simulink library "BechamoNasaOpenModels"  (R2024b)
settings: Solver=VariableStepAuto  StartTime=0.0  StopTime=10.0  RelTol=1e-3
values from neighbouring files (symbols this model uses):
  Cl_aileron_wing_1 = Cl_mat.Claileron_wing.axes1.value    [setupMavrik.m]
  Cl_aileron_wing_2 = Cl_mat.Claileron_wing.axes2.value    [setupMavrik.m]
  Cl_aileron_wing_3 = Cl_mat.Claileron_wing.axes3.value    [setupMavrik.m]
  Cl_aileron_wing_val = Cl_mat.Claileron_wing.value    [setupMavrik.m]
  Cl_elevator_tail_1 = Cl_mat.Clelevator_tail.axes1.value    [setupMavrik.m]
  Cl_elevator_tail_2 = Cl_mat.Clelevator_tail.axes2.value    [setupMavrik.m]
  Cl_elevator_tail_3 = Cl_mat.Clelevator_tail.axes3.value    [setupMavrik.m]
  Cl_elevator_tail_val = Cl_mat.Clelevator_tail.value    [setupMavrik.m]
  Cl_flap_wing_1 = Cl_mat.Clflap_wing.axes1.value    [setupMavrik.m]
  Cl_flap_wing_2 = Cl_mat.Clflap_wing.axes2.value    [setupMavrik.m]
  Cl_flap_wing_3 = Cl_mat.Clflap_wing.axes3.value    [setupMavrik.m]
  Cl_flap_wing_val = Cl_mat.Clflap_wing.value    [setupMavrik.m]
  Cl_hover_fuse_1 = Cl_mat.Clhover_fuse.axes1.value    [setupMavrik.m]
  Cl_hover_fuse_2 = Cl_mat.Clhover_fuse.axes2.value    [setupMavrik.m]
  Cl_hover_fuse_3 = Cl_mat.Clhover_fuse.axes3.value    [setupMavrik.m]
  Cl_hover_fuse_val = Cl_mat.Clhover_fuse.value    [setupMavrik.m]
  Cl_rudder_tail_1 = Cl_mat.Clrudder_tail.axes1.value    [setupMavrik.m]
  Cl_rudder_tail_2 = Cl_mat.Clrudder_tail.axes2.value    [setupMavrik.m]
  Cl_rudder_tail_3 = Cl_mat.Clrudder_tail.axes3.value    [setupMavrik.m]
  Cl_rudder_tail_val = Cl_mat.Clrudder_tail.value    [setupMavrik.m]
  Cl_tail_1 = Cl_mat.Cltail.axes1.value    [setupMavrik.m]
  Cl_tail_2 = Cl_mat.Cltail.axes2.value    [setupMavrik.m]
  Cl_tail_3 = Cl_mat.Cltail.axes3.value    [setupMavrik.m]
  Cl_tail_damp_p_1 = Cl_mat.Cltail_damp_p.axes1.value    [setupMavrik.m]
  Cl_tail_damp_p_2 = Cl_mat.Cltail_damp_p.axes2.value    [setupMavrik.m]
  Cl_tail_damp_p_3 = Cl_mat.Cltail_damp_p.axes3.value    [setupMavrik.m]
  Cl_tail_damp_p_val = Cl_mat.Cltail_damp_p.value    [setupMavrik.m]
  Cl_tail_damp_q_1 = Cl_mat.Cltail_damp_q.axes1.value    [setupMavrik.m]
  Cl_tail_damp_q_2 = Cl_mat.Cltail_damp_q.axes2.value    [setupMavrik.m]
  Cl_tail_damp_q_3 = Cl_mat.Cltail_damp_q.axes3.value    [setupMavrik.m]
  Cl_tail_damp_q_val = Cl_mat.Cltail_damp_q.value    [setupMavrik.m]
  Cl_tail_damp_r_1 = Cl_mat.Cltail_damp_r.axes1.value    [setupMavrik.m]
  Cl_tail_damp_r_2 = Cl_mat.Cltail_damp_r.axes2.value    [setupMavrik.m]
  Cl_tail_damp_r_3 = Cl_mat.Cltail_damp_r.axes3.value    [setupMavrik.m]
  Cl_tail_damp_r_val = Cl_mat.Cltail_damp_r.value    [setupMavrik.m]
  Cl_tail_val = Cl_mat.Cltail.value    [setupMavrik.m]
  Cl_wing_1 = Cl_mat.Clwing.axes1.value    [setupMavrik.m]
  Cl_wing_2 = Cl_mat.Clwing.axes2.value    [setupMavrik.m]
  Cl_wing_3 = Cl_mat.Clwing.axes3.value    [setupMavrik.m]
  Cl_wing_damp_p_1 = Cl_mat.Clwing_damp_p.axes1.value    [setupMavrik.m]
  Cl_wing_damp_p_2 = Cl_mat.Clwing_damp_p.axes2.value    [setupMavrik.m]
  Cl_wing_damp_p_3 = Cl_mat.Clwing_damp_p.axes3.value    [setupMavrik.m]
  Cl_wing_damp_p_val = Cl_mat.Clwing_damp_p.value    [setupMavrik.m]
  Cl_wing_damp_q_1 = Cl_mat.Clwing_damp_q.axes1.value    [setupMavrik.m]
  Cl_wing_damp_q_2 = Cl_mat.Clwing_damp_q.axes2.value    [setupMavrik.m]
  Cl_wing_damp_q_3 = Cl_mat.Clwing_damp_q.axes3.value    [setupMavrik.m]
  Cl_wing_damp_q_val = Cl_mat.Clwing_damp_q.value    [setupMavrik.m]
  Cl_wing_damp_r_1 = Cl_mat.Clwing_damp_r.axes1.value    [setupMavrik.m]
  Cl_wing_damp_r_2 = Cl_mat.Clwing_damp_r.axes2.value    [setupMavrik.m]
  Cl_wing_damp_r_3 = Cl_mat.Clwing_damp_r.axes3.value    [setupMavrik.m]
  Cl_wing_damp_r_val = Cl_mat.Clwing_damp_r.value    [setupMavrik.m]
  Cl_wing_val = Cl_mat.Clwing.value    [setupMavrik.m]
  Cm_aileron_wing_1 = Cm_mat.Cmaileron_wing.axes1.value    [setupMavrik.m]
  Cm_aileron_wing_2 = Cm_mat.Cmaileron_wing.axes2.value    [setupMavrik.m]
  Cm_aileron_wing_3 = Cm_mat.Cmaileron_wing.axes3.value    [setupMavrik.m]
  Cm_aileron_wing_val = Cm_mat.Cmaileron_wing.value    [setupMavrik.m]
  Cm_elevator_tail_1 = Cm_mat.Cmelevator_tail.axes1.value    [setupMavrik.m]
  Cm_elevator_tail_2 = Cm_mat.Cmelevator_tail.axes2.value    [setupMavrik.m]
  Cm_elevator_tail_3 = Cm_mat.Cmelevator_tail.axes3.value    [setupMavrik.m]
  Cm_elevator_tail_val = Cm_mat.Cmelevator_tail.value    [setupMavrik.m]
  Cm_flap_wing_1 = Cm_mat.Cmflap_wing.axes1.value    [setupMavrik.m]
  Cm_flap_wing_2 = Cm_mat.Cmflap_wing.axes2.value    [setupMavrik.m]
  Cm_flap_wing_3 = Cm_mat.Cmflap_wing.axes3.value    [setupMavrik.m]
  Cm_flap_wing_val = Cm_mat.Cmflap_wing.value    [setupMavrik.m]
  Cm_hover_fuse_1 = Cm_mat.Cmhover_fuse.axes1.value    [setupMavrik.m]
  Cm_hover_fuse_2 = Cm_mat.Cmhover_fuse.axes2.value    [setupMavrik.m]
  Cm_hover_fuse_3 = Cm_mat.Cmhover_fuse.axes3.value    [setupMavrik.m]
  Cm_hover_fuse_val = Cm_mat.Cmhover_fuse.value    [setupMavrik.m]
  Cm_rudder_tail_1 = Cm_mat.Cmrudder_tail.axes1.value    [setupMavrik.m]
  Cm_rudder_tail_2 = Cm_mat.Cmrudder_tail.axes2.value    [setupMavrik.m]
  Cm_rudder_tail_3 = Cm_mat.Cmrudder_tail.axes3.value    [setupMavrik.m]
  Cm_rudder_tail_val = Cm_mat.Cmrudder_tail.value    [setupMavrik.m]
  Cm_tail_1 = Cm_mat.Cmtail.axes1.value    [setupMavrik.m]
  Cm_tail_2 = Cm_mat.Cmtail.axes2.value    [setupMavrik.m]
  Cm_tail_3 = Cm_mat.Cmtail.axes3.value    [setupMavrik.m]
  Cm_tail_damp_p_1 = Cm_mat.Cmtail_damp_p.axes1.value    [setupMavrik.m]
  Cm_tail_damp_p_2 = Cm_mat.Cmtail_damp_p.axes2.value    [setupMavrik.m]
  Cm_tail_damp_p_3 = Cm_mat.Cmtail_damp_p.axes3.value    [setupMavrik.m]
  Cm_tail_damp_p_val = Cm_mat.Cmtail_damp_p.value    [setupMavrik.m]
  Cm_tail_damp_q_1 = Cm_mat.Cmtail_damp_q.axes1.value    [setupMavrik.m]
  Cm_tail_damp_q_2 = Cm_mat.Cmtail_damp_q.axes2.value    [setupMavrik.m]
  Cm_tail_damp_q_3 = Cm_mat.Cmtail_damp_q.axes3.value    [setupMavrik.m]
  Cm_tail_damp_q_val = Cm_mat.Cmtail_damp_q.value    [setupMavrik.m]
  Cm_tail_damp_r_1 = Cm_mat.Cmtail_damp_r.axes1.value    [setupMavrik.m]
  Cm_tail_damp_r_2 = Cm_mat.Cmtail_damp_r.axes2.value    [setupMavrik.m]
  Cm_tail_damp_r_3 = Cm_mat.Cmtail_damp_r.axes3.value    [setupMavrik.m]
  Cm_tail_damp_r_val = Cm_mat.Cmtail_damp_r.value    [setupMavrik.m]
  Cm_tail_val = Cm_mat.Cmtail.value    [setupMavrik.m]
  Cm_wing_1 = Cm_mat.Cmwing.axes1.value    [setupMavrik.m]
  Cm_wing_2 = Cm_mat.Cmwing.axes2.value    [setupMavrik.m]
  Cm_wing_3 = Cm_mat.Cmwing.axes3.value    [setupMavrik.m]
  Cm_wing_damp_p_1 = Cm_mat.Cmwing_damp_p.axes1.value    [setupMavrik.m]
  Cm_wing_damp_p_2 = Cm_mat.Cmwing_damp_p.axes2.value    [setupMavrik.m]
  Cm_wing_damp_p_3 = Cm_mat.Cmwing_damp_p.axes3.value    [setupMavrik.m]
  Cm_wing_damp_p_val = Cm_mat.Cmwing_damp_p.value    [setupMavrik.m]
  Cm_wing_damp_q_1 = Cm_mat.Cmwing_damp_q.axes1.value    [setupMavrik.m]
  Cm_wing_damp_q_2 = Cm_mat.Cmwing_damp_q.axes2.value    [setupMavrik.m]
  Cm_wing_damp_q_3 = Cm_mat.Cmwing_damp_q.axes3.value    [setupMavrik.m]
  Cm_wing_damp_q_val = Cm_mat.Cmwing_damp_q.value    [setupMavrik.m]
  Cm_wing_damp_r_1 = Cm_mat.Cmwing_damp_r.axes1.value    [setupMavrik.m]
  Cm_wing_damp_r_2 = Cm_mat.Cmwing_damp_r.axes2.value    [setupMavrik.m]
  Cm_wing_damp_r_3 = Cm_mat.Cmwing_damp_r.axes3.value    [setupMavrik.m]
  Cm_wing_damp_r_val = Cm_mat.Cmwing_damp_r.value    [setupMavrik.m]
  Cm_wing_val = Cm_mat.Cmwing.value    [setupMavrik.m]
  Cn_aileron_wing_1 = Cn_mat.Cnaileron_wing.axes1.value    [setupMavrik.m]
  Cn_aileron_wing_2 = Cn_mat.Cnaileron_wing.axes2.value    [setupMavrik.m]
  Cn_aileron_wing_3 = Cn_mat.Cnaileron_wing.axes3.value    [setupMavrik.m]
  Cn_aileron_wing_val = Cn_mat.Cnaileron_wing.value    [setupMavrik.m]
  Cn_elevator_tail_1 = Cn_mat.Cnelevator_tail.axes1.value    [setupMavrik.m]
  Cn_elevator_tail_2 = Cn_mat.Cnelevator_tail.axes2.value    [setupMavrik.m]
  Cn_elevator_tail_3 = Cn_mat.Cnelevator_tail.axes3.value    [setupMavrik.m]
  Cn_elevator_tail_val = Cn_mat.Cnelevator_tail.value    [setupMavrik.m]
  Cn_flap_wing_1 = Cn_mat.Cnflap_wing.axes1.value    [setupMavrik.m]
  Cn_flap_wing_2 = Cn_mat.Cnflap_wing.axes2.value    [setupMavrik.m]
  Cn_flap_wing_3 = Cn_mat.Cnflap_wing.axes3.value    [setupMavrik.m]
  Cn_flap_wing_val = Cn_mat.Cnflap_wing.value    [setupMavrik.m]
  Cn_hover_fuse_1 = Cn_mat.Cnhover_fuse.axes1.value    [setupMavrik.m]
  Cn_hover_fuse_2 = Cn_mat.Cnhover_fuse.axes2.value    [setupMavrik.m]
  Cn_hover_fuse_3 = Cn_mat.Cnhover_fuse.axes3.value    [setupMavrik.m]
  Cn_hover_fuse_val = Cn_mat.Cnhover_fuse.value    [setupMavrik.m]
  ... (+319 more)
libraries: matrix_library x15, sharedtransform x2, $bdroot x1, shared6dof x1
(part 4 of 19)

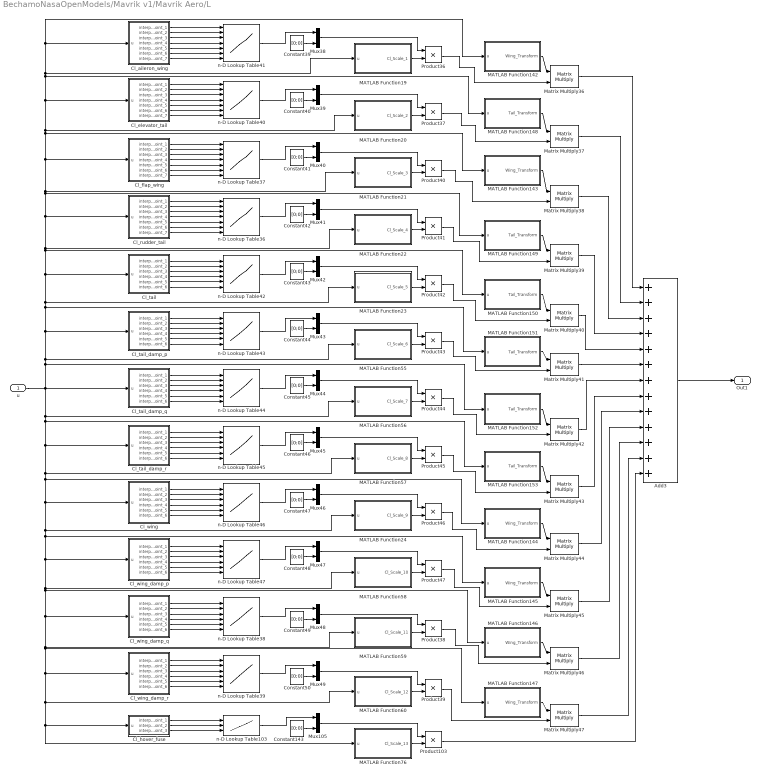
== system BechamoNasaOpenModels/Mavrik v1/Mavrik Aero/L ==
  u : Inport
  Add3 : Sum  Inputs=+++++++++++++
  Cl_aileron_wing : MATLAB Function  TreatAsAtomicUnit=on
  Cl_elevator_tail : MATLAB Function  TreatAsAtomicUnit=on
  Cl_flap_wing : MATLAB Function  TreatAsAtomicUnit=on
  Cl_hover_fuse : MATLAB Function  TreatAsAtomicUnit=on
  Cl_rudder_tail : MATLAB Function  TreatAsAtomicUnit=on
  Cl_tail : MATLAB Function  TreatAsAtomicUnit=on
  Cl_tail_damp_p : MATLAB Function  TreatAsAtomicUnit=on
  Cl_tail_damp_q : MATLAB Function  TreatAsAtomicUnit=on
  Cl_tail_damp_r : MATLAB Function  TreatAsAtomicUnit=on
  Cl_wing : MATLAB Function  TreatAsAtomicUnit=on
  Cl_wing_damp_p : MATLAB Function  TreatAsAtomicUnit=on
  Cl_wing_damp_q : MATLAB Function  TreatAsAtomicUnit=on
  Cl_wing_damp_r : MATLAB Function  TreatAsAtomicUnit=on
  Constant{39..50,143} (13 alike) : Constant  Value=[0;0]
  MATLAB Function142 : MATLAB Function  TreatAsAtomicUnit=on
  MATLAB Function143 : MATLAB Function  TreatAsAtomicUnit=on
  MATLAB Function144 : MATLAB Function  TreatAsAtomicUnit=on
  MATLAB Function145 : MATLAB Function  TreatAsAtomicUnit=on
  MATLAB Function146 : MATLAB Function  TreatAsAtomicUnit=on
  MATLAB Function147 : MATLAB Function  TreatAsAtomicUnit=on
  MATLAB Function148 : MATLAB Function  TreatAsAtomicUnit=on
  MATLAB Function149 : MATLAB Function  TreatAsAtomicUnit=on
  MATLAB Function150 : MATLAB Function  TreatAsAtomicUnit=on
  MATLAB Function151 : MATLAB Function  TreatAsAtomicUnit=on
  MATLAB Function152 : MATLAB Function  TreatAsAtomicUnit=on
  MATLAB Function153 : MATLAB Function  TreatAsAtomicUnit=on
  MATLAB Function19 : MATLAB Function  TreatAsAtomicUnit=on
  MATLAB Function20 : MATLAB Function  TreatAsAtomicUnit=on
  MATLAB Function21 : MATLAB Function  TreatAsAtomicUnit=on
  MATLAB Function22 : MATLAB Function  TreatAsAtomicUnit=on
  MATLAB Function23 : MATLAB Function  TreatAsAtomicUnit=on
  MATLAB Function24 : MATLAB Function  TreatAsAtomicUnit=on
  MATLAB Function55 : MATLAB Function  TreatAsAtomicUnit=on
  MATLAB Function56 : MATLAB Function  TreatAsAtomicUnit=on
  MATLAB Function57 : MATLAB Function  TreatAsAtomicUnit=on
  MATLAB Function58 : MATLAB Function  TreatAsAtomicUnit=on
  MATLAB Function59 : MATLAB Function  TreatAsAtomicUnit=on
  MATLAB Function60 : MATLAB Function  TreatAsAtomicUnit=on
  MATLAB Function76 : MATLAB Function  TreatAsAtomicUnit=on
  Matrix Multiply{36..47} (12 alike) : Product  Multiplication=Matrix(*)
  Mux{38..49,105} (13 alike) : Mux  Inputs=2
  Product{36..47,103} (13 alike) : Product
  n-D Lookup Table103 : Lookup_n-D  NumberOfTableDimensions=3  BreakpointsForDimension1=Cl_hover_fuse_1  BreakpointsForDimension2=Cl_hover_fuse_2  BreakpointsForDimension3=Cl_hover_fuse_3  BreakpointsForDimension4=CX_wing_damp_r_4  BreakpointsForDimension5=CX_wing_damp_r_5  BreakpointsForDimension6=CX_wing_damp_r_6  BreakpointsForDimension7=CX_flap_wing_7  Table=Cl_hover_fuse_val  InternalRulePriority=Speed  OutDataTypeStr=Inherit: Inherit via back propagation  RndMeth=Simplest
      settings: InputPortMap=u0,u1,u2
  n-D Lookup Table36 : Lookup_n-D  NumberOfTableDimensions=7  BreakpointsForDimension1=Cl_rudder_tail_1  BreakpointsForDimension2=Cl_rudder_tail_2  BreakpointsForDimension3=Cl_rudder_tail_3  BreakpointsForDimension4=Cl_rudder_tail_4  BreakpointsForDimension5=Cl_rudder_tail_5  BreakpointsForDimension6=Cl_rudder_tail_6  BreakpointsForDimension7=Cl_rudder_tail_7  Table=Cl_rudder_tail_val  InternalRulePriority=Speed  OutDataTypeStr=Inherit: Inherit via back propagation  RndMeth=Simplest
      settings: InputPortMap=u0,u1,u2,u3,u4,u5,u6
  n-D Lookup Table37 : Lookup_n-D  NumberOfTableDimensions=7  BreakpointsForDimension1=Cl_flap_wing_1  BreakpointsForDimension2=Cl_flap_wing_2  BreakpointsForDimension3=Cl_flap_wing_3  BreakpointsForDimension4=Cl_flap_wing_4  BreakpointsForDimension5=Cl_flap_wing_5  BreakpointsForDimension6=Cl_flap_wing_6  BreakpointsForDimension7=Cl_flap_wing_7  Table=Cl_flap_wing_val  InternalRulePriority=Speed  OutDataTypeStr=Inherit: Inherit via back propagation  RndMeth=Simplest
      settings: InputPortMap=u0,u1,u2,u3,u4,u5,u6
  n-D Lookup Table38 : Lookup_n-D  NumberOfTableDimensions=6  BreakpointsForDimension1=Cl_wing_damp_q_1  BreakpointsForDimension2=Cl_wing_damp_q_2  BreakpointsForDimension3=Cl_wing_damp_q_3  BreakpointsForDimension4=Cl_wing_damp_q_4  BreakpointsForDimension5=Cl_wing_damp_q_5  BreakpointsForDimension6=Cl_wing_damp_q_6  BreakpointsForDimension7=CX_flap_wing_7  Table=Cl_wing_damp_q_val  InternalRulePriority=Speed  OutDataTypeStr=Inherit: Inherit via back propagation  RndMeth=Simplest
      settings: InputPortMap=u0,u1,u2,u3,u4,u5
  n-D Lookup Table39 : Lookup_n-D  NumberOfTableDimensions=6  BreakpointsForDimension1=Cl_wing_damp_r_1  BreakpointsForDimension2=Cl_wing_damp_r_2  BreakpointsForDimension3=Cl_wing_damp_r_3  BreakpointsForDimension4=Cl_wing_damp_r_4  BreakpointsForDimension5=Cl_wing_damp_r_5  BreakpointsForDimension6=Cl_wing_damp_r_6  BreakpointsForDimension7=CX_flap_wing_7  Table=Cl_wing_damp_r_val  InternalRulePriority=Speed  OutDataTypeStr=Inherit: Inherit via back propagation  RndMeth=Simplest
      settings: InputPortMap=u0,u1,u2,u3,u4,u5
  n-D Lookup Table40 : Lookup_n-D  NumberOfTableDimensions=7  BreakpointsForDimension1=Cl_elevator_tail_1  BreakpointsForDimension2=Cl_elevator_tail_2  BreakpointsForDimension3=Cl_elevator_tail_3  BreakpointsForDimension4=Cl_elevator_tail_4  BreakpointsForDimension5=Cl_elevator_tail_5  BreakpointsForDimension6=Cl_elevator_tail_6  BreakpointsForDimension7=Cl_elevator_tail_7  Table=Cl_elevator_tail_val  InternalRulePriority=Speed  OutDataTypeStr=Inherit: Inherit via back propagation  RndMeth=Simplest
      settings: InputPortMap=u0,u1,u2,u3,u4,u5,u6
  n-D Lookup Table41 : Lookup_n-D  NumberOfTableDimensions=7  BreakpointsForDimension1=Cl_aileron_wing_1  BreakpointsForDimension2=Cl_aileron_wing_2  BreakpointsForDimension3=Cl_aileron_wing_3  BreakpointsForDimension4=Cl_aileron_wing_4  BreakpointsForDimension5=Cl_aileron_wing_5  BreakpointsForDimension6=Cl_aileron_wing_6  BreakpointsForDimension7=Cl_aileron_wing_7  Table=Cl_aileron_wing_val  InternalRulePriority=Speed  OutDataTypeStr=Inherit: Inherit via back propagation  RndMeth=Simplest
      settings: InputPortMap=u0,u1,u2,u3,u4,u5,u6
  n-D Lookup Table42 : Lookup_n-D  NumberOfTableDimensions=6  BreakpointsForDimension1=Cl_tail_1  BreakpointsForDimension2=Cl_tail_2  BreakpointsForDimension3=Cl_tail_3  BreakpointsForDimension4=Cl_tail_4  BreakpointsForDimension5=Cl_tail_5  BreakpointsForDimension6=Cl_tail_6  BreakpointsForDimension7=CX_tail_7  Table=Cl_tail_val  InternalRulePriority=Speed  OutDataTypeStr=Inherit: Inherit via back propagation  RndMeth=Simplest
      settings: InputPortMap=u0,u1,u2,u3,u4,u5
  n-D Lookup Table43 : Lookup_n-D  NumberOfTableDimensions=6  BreakpointsForDimension1=Cl_tail_damp_p_1  BreakpointsForDimension2=Cl_tail_damp_p_2  BreakpointsForDimension3=Cl_tail_damp_p_3  BreakpointsForDimension4=Cl_tail_damp_p_4  BreakpointsForDimension5=Cl_tail_damp_p_5  BreakpointsForDimension6=Cl_tail_damp_p_6  BreakpointsForDimension7=CX_tail_7  Table=Cl_tail_damp_p_val  InternalRulePriority=Speed  OutDataTypeStr=Inherit: Inherit via back propagation  RndMeth=Simplest
      settings: InputPortMap=u0,u1,u2,u3,u4,u5
  n-D Lookup Table44 : Lookup_n-D  NumberOfTableDimensions=6  BreakpointsForDimension1=Cl_tail_damp_q_1  BreakpointsForDimension2=Cl_tail_damp_q_2  BreakpointsForDimension3=Cl_tail_damp_q_3  BreakpointsForDimension4=Cl_tail_damp_q_4  BreakpointsForDimension5=Cl_tail_damp_q_5  BreakpointsForDimension6=Cl_tail_damp_q_6  BreakpointsForDimension7=CX_tail_7  Table=Cl_tail_damp_q_val  InternalRulePriority=Speed  OutDataTypeStr=Inherit: Inherit via back propagation  RndMeth=Simplest
      settings: InputPortMap=u0,u1,u2,u3,u4,u5
  n-D Lookup Table45 : Lookup_n-D  NumberOfTableDimensions=6  BreakpointsForDimension1=Cl_tail_damp_r_1  BreakpointsForDimension2=Cl_tail_damp_r_2  BreakpointsForDimension3=Cl_tail_damp_r_3  BreakpointsForDimension4=Cl_tail_damp_r_4  BreakpointsForDimension5=Cl_tail_damp_r_5  BreakpointsForDimension6=Cl_tail_damp_r_6  BreakpointsForDimension7=CX_tail_7  Table=Cl_tail_damp_r_val  InternalRulePriority=Speed  OutDataTypeStr=Inherit: Inherit via back propagation  RndMeth=Simplest
      settings: InputPortMap=u0,u1,u2,u3,u4,u5
  n-D Lookup Table46 : Lookup_n-D  NumberOfTableDimensions=6  BreakpointsForDimension1=Cl_wing_1  BreakpointsForDimension2=Cl_wing_2  BreakpointsForDimension3=Cl_wing_3  BreakpointsForDimension4=Cl_wing_4  BreakpointsForDimension5=Cl_wing_5  BreakpointsForDimension6=Cl_wing_6  BreakpointsForDimension7=CX_flap_wing_7  Table=Cl_wing_val  InternalRulePriority=Speed  OutDataTypeStr=Inherit: Inherit via back propagation  RndMeth=Simplest
      settings: InputPortMap=u0,u1,u2,u3,u4,u5
  n-D Lookup Table47 : Lookup_n-D  NumberOfTableDimensions=6  BreakpointsForDimension1=Cl_wing_damp_p_1  BreakpointsForDimension2=Cl_wing_damp_p_2  BreakpointsForDimension3=Cl_wing_damp_p_3  BreakpointsForDimension4=Cl_wing_damp_p_4  BreakpointsForDimension5=Cl_wing_damp_p_5  BreakpointsForDimension6=Cl_wing_damp_p_6  BreakpointsForDimension7=CX_flap_wing_7  Table=Cl_wing_damp_p_val  InternalRulePriority=Speed  OutDataTypeStr=Inherit: Inherit via back propagation  RndMeth=Simplest
      settings: InputPortMap=u0,u1,u2,u3,u4,u5
  Out1 : Outport
  wires:
  Cl_hover_fuse/3(interp_point_3) -> n-D Lookup Table103/3
  Cl_wing_damp_q/1(interp_point_1) -> n-D Lookup Table38/1
  Add3/1 -> Out1/1
  Cl_wing/3(interp_point_3) -> n-D Lookup Table46/3
  MATLAB Function57/1(Cl_Scale_8) -> Product45/2
  Cl_tail_damp_q/3(interp_point_3) -> n-D Lookup Table44/3
  Matrix Multiply46/1 -> Add3/11
  Cl_elevator_tail/5(interp_point_5) -> n-D Lookup Table40/5
  MATLAB Function153/1(Tail_Transform) -> Matrix Multiply43/1
  Matrix Multiply40/1 -> Add3/5
  Cl_rudder_tail/4(interp_point_4) -> n-D Lookup Table36/4
  Cl_tail_damp_r/1(interp_point_1) -> n-D Lookup Table45/1
  Matrix Multiply38/1 -> Add3/3
  Matrix Multiply37/1 -> Add3/2
  Cl_tail_damp_p/5(interp_point_5) -> n-D Lookup Table43/5
  Mux48/1 -> Product38/1
  Cl_wing_damp_p/6(interp_point_6) -> n-D Lookup Table47/6
  Cl_wing_damp_q/4(interp_point_4) -> n-D Lookup Table38/4
  MATLAB Function21/1(Cl_Scale_3) -> Product40/2
  Cl_wing_damp_p/5(interp_point_5) -> n-D Lookup Table47/5
  Mux44/1 -> Product44/1
  Matrix Multiply36/1 -> Add3/1
  Cl_rudder_tail/5(interp_point_5) -> n-D Lookup Table36/5
  Product44/1 -> Matrix Multiply42/2
  Mux41/1 -> Product41/1
  Cl_elevator_tail/4(interp_point_4) -> n-D Lookup Table40/4
  Cl_rudder_tail/2(interp_point_2) -> n-D Lookup Table36/2
  Cl_wing_damp_p/3(interp_point_3) -> n-D Lookup Table47/3
  Cl_elevator_tail/2(interp_point_2) -> n-D Lookup Table40/2
  Mux42/1 -> Product42/1
  Cl_tail/3(interp_point_3) -> n-D Lookup Table42/3
  Cl_wing/5(interp_point_5) -> n-D Lookup Table46/5
  Cl_tail_damp_r/5(interp_point_5) -> n-D Lookup Table45/5
  Cl_wing/2(interp_point_2) -> n-D Lookup Table46/2
  Cl_tail_damp_q/4(interp_point_4) -> n-D Lookup Table44/4
  Cl_flap_wing/3(interp_point_3) -> n-D Lookup Table37/3
  Mux47/1 -> Product47/1
  Cl_tail/5(interp_point_5) -> n-D Lookup Table42/5
  Product103/1 -> Add3/13
  Cl_elevator_tail/1(interp_point_1) -> n-D Lookup Table40/1
  Cl_tail_damp_q/1(interp_point_1) -> n-D Lookup Table44/1
  Constant47/1 -> Mux46/2
  Cl_wing_damp_r/3(interp_point_3) -> n-D Lookup Table39/3
  Cl_wing_damp_r/4(interp_point_4) -> n-D Lookup Table39/4
  Cl_tail_damp_q/2(interp_point_2) -> n-D Lookup Table44/2
  MATLAB Function24/1(Cl_Scale_9) -> Product46/2
  Cl_tail/6(interp_point_6) -> n-D Lookup Table42/6
  Cl_rudder_tail/3(interp_point_3) -> n-D Lookup Table36/3
  MATLAB Function142/1(Wing_Transform) -> Matrix Multiply36/1
  Cl_hover_fuse/1(interp_point_1) -> n-D Lookup Table103/1
  Cl_wing/1(interp_point_1) -> n-D Lookup Table46/1
  Cl_wing_damp_q/6(interp_point_6) -> n-D Lookup Table38/6
  Cl_rudder_tail/7(interp_point_7) -> n-D Lookup Table36/7
  Cl_aileron_wing/1(interp_point_1) -> n-D Lookup Table41/1
  Cl_wing/6(interp_point_6) -> n-D Lookup Table46/6
  n-D Lookup Table44/1 -> Mux44/1
  Cl_elevator_tail/7(interp_point_7) -> n-D Lookup Table40/7
  Cl_tail_damp_p/6(interp_point_6) -> n-D Lookup Table43/6
  Constant42/1 -> Mux41/2
  u/1 -> MATLAB Function56/1(u), MATLAB Function153/1(u), Cl_tail_damp_r/1(u), MATLAB Function57/1(u), MATLAB Function144/1(u), Cl_wing/1(u), MATLAB Function24/1(u), MATLAB Function145/1(u), Cl_wing_damp_p/1(u), MATLAB Function58/1(u), MATLAB Function146/1(u), Cl_wing_damp_q/1(u), MATLAB Function59/1(u), Cl_wing_damp_r/1(u), MATLAB Function60/1(u), Cl_hover_fuse/1(u), MATLAB Function76/1(u), MATLAB Function147/1(u), MATLAB Function152/1(u), MATLAB Function55/1(u), Cl_tail_damp_p/1(u), MATLAB Function151/1(u), MATLAB Function23/1(u), Cl_tail/1(u), MATLAB Function150/1(u), MATLAB Function22/1(u), Cl_rudder_tail/1(u), MATLAB Function149/1(u), MATLAB Function21/1(u), Cl_flap_wing/1(u), MATLAB Function143/1(u), MATLAB Function20/1(u), Cl_elevator_tail/1(u), MATLAB Function148/1(u), Cl_aileron_wing/1(u), MATLAB Function142/1(u), MATLAB Function19/1(u), Cl_tail_damp_q/1(u)
  Cl_wing_damp_r/5(interp_point_5) -> n-D Lookup Table39/5
  Cl_hover_fuse/2(interp_point_2) -> n-D Lookup Table103/2
  Cl_aileron_wing/3(interp_point_3) -> n-D Lookup Table41/3
  MATLAB Function147/1(Wing_Transform) -> Matrix Multiply47/1
  Cl_flap_wing/1(interp_point_1) -> n-D Lookup Table37/1
  Constant41/1 -> Mux40/2
  Cl_tail_damp_p/3(interp_point_3) -> n-D Lookup Table43/3
  Cl_tail_damp_p/4(interp_point_4) -> n-D Lookup Table43/4
  n-D Lookup Table103/1 -> Mux105/1
  Cl_tail_damp_r/4(interp_point_4) -> n-D Lookup Table45/4
  n-D Lookup Table46/1 -> Mux46/1
  Cl_tail_damp_q/5(interp_point_5) -> n-D Lookup Table44/5
  Cl_tail_damp_r/6(interp_point_6) -> n-D Lookup Table45/6
  Cl_flap_wing/5(interp_point_5) -> n-D Lookup Table37/5
  Cl_tail_damp_r/2(interp_point_2) -> n-D Lookup Table45/2
  Cl_wing/4(interp_point_4) -> n-D Lookup Table46/4
  Constant50/1 -> Mux49/2
  MATLAB Function60/1(Cl_Scale_12) -> Product39/2
  MATLAB Function76/1(Cl_Scale_13) -> Product103/2
  Cl_wing_damp_p/2(interp_point_2) -> n-D Lookup Table47/2
  Cl_wing_damp_p/1(interp_point_1) -> n-D Lookup Table47/1
  Matrix Multiply39/1 -> Add3/4
  MATLAB Function59/1(Cl_Scale_11) -> Product38/2
  Cl_aileron_wing/4(interp_point_4) -> n-D Lookup Table41/4
  Cl_wing_damp_r/1(interp_point_1) -> n-D Lookup Table39/1
  Cl_wing_damp_r/6(interp_point_6) -> n-D Lookup Table39/6
  Cl_tail/4(interp_point_4) -> n-D Lookup Table42/4
  MATLAB Function145/1(Wing_Transform) -> Matrix Multiply45/1
  MATLAB Function144/1(Wing_Transform) -> Matrix Multiply44/1
  Cl_flap_wing/6(interp_point_6) -> n-D Lookup Table37/6
  Cl_flap_wing/4(interp_point_4) -> n-D Lookup Table37/4
  Mux45/1 -> Product45/1
  Cl_tail_damp_q/6(interp_point_6) -> n-D Lookup Table44/6
  n-D Lookup Table42/1 -> Mux42/1
  MATLAB Function151/1(Tail_Transform) -> Matrix Multiply41/1
  Matrix Multiply45/1 -> Add3/10
  Cl_tail/2(interp_point_2) -> n-D Lookup Table42/2
  Constant143/1 -> Mux105/2
  Mux39/1 -> Product37/1
  Product42/1 -> Matrix Multiply40/2
  Cl_flap_wing/2(interp_point_2) -> n-D Lookup Table37/2
  Cl_tail/1(interp_point_1) -> n-D Lookup Table42/1
  Product38/1 -> Matrix Multiply46/2
  Cl_aileron_wing/7(interp_point_7) -> n-D Lookup Table41/7
  MATLAB Function20/1(Cl_Scale_2) -> Product37/2
  Product41/1 -> Matrix Multiply39/2
  MATLAB Function146/1(Wing_Transform) -> Matrix Multiply46/1
  Cl_wing_damp_q/5(interp_point_5) -> n-D Lookup Table38/5
  MATLAB Function23/1(Cl_Scale_5) -> Product42/2
  MATLAB Function148/1(Tail_Transform) -> Matrix Multiply37/1
  n-D Lookup Table39/1 -> Mux49/1
  Product46/1 -> Matrix Multiply44/2
  Matrix Multiply44/1 -> Add3/9
  Matrix Multiply47/1 -> Add3/12
  Matrix Multiply41/1 -> Add3/6
  Matrix Multiply42/1 -> Add3/7
  n-D Lookup Table43/1 -> Mux43/1
  n-D Lookup Table41/1 -> Mux38/1
  Constant44/1 -> Mux43/2
  n-D Lookup Table45/1 -> Mux45/1
  Constant46/1 -> Mux45/2
  Constant49/1 -> Mux48/2
  n-D Lookup Table47/1 -> Mux47/1
  Constant48/1 -> Mux47/2
  n-D Lookup Table38/1 -> Mux48/1
  Cl_wing_damp_q/2(interp_point_2) -> n-D Lookup Table38/2
  Mux38/1 -> Product36/1
  MATLAB Function149/1(Tail_Transform) -> Matrix Multiply39/1
  n-D Lookup Table40/1 -> Mux39/1
  n-D Lookup Table37/1 -> Mux40/1
  Product39/1 -> Matrix Multiply47/2
  Cl_wing_damp_q/3(interp_point_3) -> n-D Lookup Table38/3
  Cl_tail_damp_p/2(interp_point_2) -> n-D Lookup Table43/2
  Constant39/1 -> Mux38/2
  MATLAB Function56/1(Cl_Scale_7) -> Product44/2
  Constant40/1 -> Mux39/2
  MATLAB Function55/1(Cl_Scale_6) -> Product43/2
  MATLAB Function58/1(Cl_Scale_10) -> Product47/2
  Cl_flap_wing/7(interp_point_7) -> n-D Lookup Table37/7
  Cl_aileron_wing/2(interp_point_2) -> n-D Lookup Table41/2
  Cl_tail_damp_p/1(interp_point_1) -> n-D Lookup Table43/1
  Cl_elevator_tail/6(interp_point_6) -> n-D Lookup Table40/6
  Matrix Multiply43/1 -> Add3/8
  Cl_aileron_wing/6(interp_point_6) -> n-D Lookup Table41/6
  Mux49/1 -> Product39/1
  Mux46/1 -> Product46/1
  Cl_wing_damp_r/2(interp_point_2) -> n-D Lookup Table39/2
  Constant45/1 -> Mux44/2
  Mux40/1 -> Product40/1
  Cl_rudder_tail/6(interp_point_6) -> n-D Lookup Table36/6
  Cl_elevator_tail/3(interp_point_3) -> n-D Lookup Table40/3
  MATLAB Function19/1(Cl_Scale_1) -> Product36/2
  MATLAB Function143/1(Wing_Transform) -> Matrix Multiply38/1
  Mux43/1 -> Product43/1
  MATLAB Function152/1(Tail_Transform) -> Matrix Multiply42/1
  MATLAB Function22/1(Cl_Scale_4) -> Product41/2
  n-D Lookup Table36/1 -> Mux41/1
  Cl_wing_damp_p/4(interp_point_4) -> n-D Lookup Table47/4
  Constant43/1 -> Mux42/2
  Cl_tail_damp_r/3(interp_point_3) -> n-D Lookup Table45/3
  Product36/1 -> Matrix Multiply36/2
  Product37/1 -> Matrix Multiply37/2
  Product43/1 -> Matrix Multiply41/2
  Product40/1 -> Matrix Multiply38/2
  Product47/1 -> Matrix Multiply45/2
  Product45/1 -> Matrix Multiply43/2
  Mux105/1 -> Product103/1
  Cl_rudder_tail/1(interp_point_1) -> n-D Lookup Table36/1
  Cl_aileron_wing/5(interp_point_5) -> n-D Lookup Table41/5
  MATLAB Function150/1(Tail_Transform) -> Matrix Multiply40/1

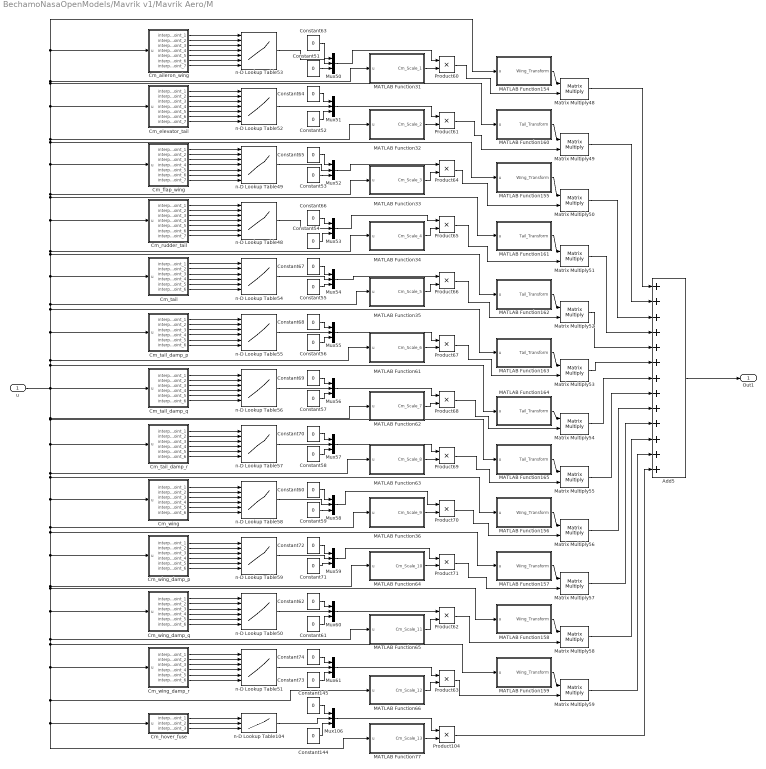
== system BechamoNasaOpenModels/Mavrik v1/Mavrik Aero/M ==
  u : Inport
  Add5 : Sum  Inputs=+++++++++++++
  Cm_aileron_wing : MATLAB Function  TreatAsAtomicUnit=on
  Cm_elevator_tail : MATLAB Function  TreatAsAtomicUnit=on
  Cm_flap_wing : MATLAB Function  TreatAsAtomicUnit=on
  Cm_hover_fuse : MATLAB Function  TreatAsAtomicUnit=on
  Cm_rudder_tail : MATLAB Function  TreatAsAtomicUnit=on
  Cm_tail : MATLAB Function  TreatAsAtomicUnit=on
  Cm_tail_damp_p : MATLAB Function  TreatAsAtomicUnit=on
  Cm_tail_damp_q : MATLAB Function  TreatAsAtomicUnit=on
  Cm_tail_damp_r : MATLAB Function  TreatAsAtomicUnit=on
  Cm_wing : MATLAB Function  TreatAsAtomicUnit=on
  Cm_wing_damp_p : MATLAB Function  TreatAsAtomicUnit=on
  Cm_wing_damp_q : MATLAB Function  TreatAsAtomicUnit=on
  Cm_wing_damp_r : MATLAB Function  TreatAsAtomicUnit=on
  Constant{51..74,144..145} (26 alike) : Constant  Value=0
  MATLAB Function154 : MATLAB Function  TreatAsAtomicUnit=on
  MATLAB Function155 : MATLAB Function  TreatAsAtomicUnit=on
  MATLAB Function156 : MATLAB Function  TreatAsAtomicUnit=on
  MATLAB Function157 : MATLAB Function  TreatAsAtomicUnit=on
  MATLAB Function158 : MATLAB Function  TreatAsAtomicUnit=on
  MATLAB Function159 : MATLAB Function  TreatAsAtomicUnit=on
  MATLAB Function160 : MATLAB Function  TreatAsAtomicUnit=on
  MATLAB Function161 : MATLAB Function  TreatAsAtomicUnit=on
  MATLAB Function162 : MATLAB Function  TreatAsAtomicUnit=on
  MATLAB Function163 : MATLAB Function  TreatAsAtomicUnit=on
  MATLAB Function164 : MATLAB Function  TreatAsAtomicUnit=on
  MATLAB Function165 : MATLAB Function  TreatAsAtomicUnit=on
  MATLAB Function31 : MATLAB Function  TreatAsAtomicUnit=on
  MATLAB Function32 : MATLAB Function  TreatAsAtomicUnit=on
  MATLAB Function33 : MATLAB Function  TreatAsAtomicUnit=on
  MATLAB Function34 : MATLAB Function  TreatAsAtomicUnit=on
  MATLAB Function35 : MATLAB Function  TreatAsAtomicUnit=on
  MATLAB Function36 : MATLAB Function  TreatAsAtomicUnit=on
  MATLAB Function61 : MATLAB Function  TreatAsAtomicUnit=on
  MATLAB Function62 : MATLAB Function  TreatAsAtomicUnit=on
  MATLAB Function63 : MATLAB Function  TreatAsAtomicUnit=on
  MATLAB Function64 : MATLAB Function  TreatAsAtomicUnit=on
  MATLAB Function65 : MATLAB Function  TreatAsAtomicUnit=on
  MATLAB Function66 : MATLAB Function  TreatAsAtomicUnit=on
  MATLAB Function77 : MATLAB Function  TreatAsAtomicUnit=on
  Matrix Multiply{48..59} (12 alike) : Product  Multiplication=Matrix(*)
  Mux{50..61,106} (13 alike) : Mux  Inputs=3
  Product{60..71,104} (13 alike) : Product
  n-D Lookup Table104 : Lookup_n-D  NumberOfTableDimensions=3  BreakpointsForDimension1=Cm_hover_fuse_1  BreakpointsForDimension2=Cm_hover_fuse_2  BreakpointsForDimension3=Cm_hover_fuse_3  BreakpointsForDimension4=CX_wing_damp_r_4  BreakpointsForDimension5=CX_wing_damp_r_5  BreakpointsForDimension6=CX_wing_damp_r_6  BreakpointsForDimension7=CX_flap_wing_7  Table=Cm_hover_fuse_val  InternalRulePriority=Speed  OutDataTypeStr=Inherit: Inherit via back propagation  RndMeth=Simplest
      settings: InputPortMap=u0,u1,u2
  n-D Lookup Table48 : Lookup_n-D  NumberOfTableDimensions=7  BreakpointsForDimension1=Cm_rudder_tail_1  BreakpointsForDimension2=Cm_rudder_tail_2  BreakpointsForDimension3=Cm_rudder_tail_3  BreakpointsForDimension4=Cm_rudder_tail_4  BreakpointsForDimension5=Cm_rudder_tail_5  BreakpointsForDimension6=Cm_rudder_tail_6  BreakpointsForDimension7=Cm_rudder_tail_7  Table=Cm_rudder_tail_val  InternalRulePriority=Speed  OutDataTypeStr=Inherit: Inherit via back propagation  RndMeth=Simplest
      settings: InputPortMap=u0,u1,u2,u3,u4,u5,u6
  n-D Lookup Table49 : Lookup_n-D  NumberOfTableDimensions=7  BreakpointsForDimension1=Cm_flap_wing_1  BreakpointsForDimension2=Cm_flap_wing_2  BreakpointsForDimension3=Cm_flap_wing_3  BreakpointsForDimension4=Cm_flap_wing_4  BreakpointsForDimension5=Cm_flap_wing_5  BreakpointsForDimension6=Cm_flap_wing_6  BreakpointsForDimension7=Cm_flap_wing_7  Table=Cm_flap_wing_val  InternalRulePriority=Speed  OutDataTypeStr=Inherit: Inherit via back propagation  RndMeth=Simplest
      settings: InputPortMap=u0,u1,u2,u3,u4,u5,u6
  n-D Lookup Table50 : Lookup_n-D  NumberOfTableDimensions=6  BreakpointsForDimension1=Cm_wing_damp_q_1  BreakpointsForDimension2=Cm_wing_damp_q_2  BreakpointsForDimension3=Cm_wing_damp_q_3  BreakpointsForDimension4=Cm_wing_damp_q_4  BreakpointsForDimension5=Cm_wing_damp_q_5  BreakpointsForDimension6=Cm_wing_damp_q_6  BreakpointsForDimension7=CX_flap_wing_7  Table=Cm_wing_damp_q_val  InternalRulePriority=Speed  OutDataTypeStr=Inherit: Inherit via back propagation  RndMeth=Simplest
      settings: InputPortMap=u0,u1,u2,u3,u4,u5
  n-D Lookup Table51 : Lookup_n-D  NumberOfTableDimensions=6  BreakpointsForDimension1=Cm_wing_damp_r_1  BreakpointsForDimension2=Cm_wing_damp_r_2  BreakpointsForDimension3=Cm_wing_damp_r_3  BreakpointsForDimension4=Cm_wing_damp_r_4  BreakpointsForDimension5=Cm_wing_damp_r_5  BreakpointsForDimension6=Cm_wing_damp_r_6  BreakpointsForDimension7=CX_flap_wing_7  Table=Cm_wing_damp_r_val  InternalRulePriority=Speed  OutDataTypeStr=Inherit: Inherit via back propagation  RndMeth=Simplest
      settings: InputPortMap=u0,u1,u2,u3,u4,u5
  n-D Lookup Table52 : Lookup_n-D  NumberOfTableDimensions=7  BreakpointsForDimension1=Cm_elevator_tail_1  BreakpointsForDimension2=Cm_elevator_tail_2  BreakpointsForDimension3=Cm_elevator_tail_3  BreakpointsForDimension4=Cm_elevator_tail_4  BreakpointsForDimension5=Cm_elevator_tail_5  BreakpointsForDimension6=Cm_elevator_tail_6  BreakpointsForDimension7=Cm_elevator_tail_7  Table=Cm_elevator_tail_val  InternalRulePriority=Speed  OutDataTypeStr=Inherit: Inherit via back propagation  RndMeth=Simplest
      settings: InputPortMap=u0,u1,u2,u3,u4,u5,u6
  n-D Lookup Table53 : Lookup_n-D  NumberOfTableDimensions=7  BreakpointsForDimension1=Cm_aileron_wing_1  BreakpointsForDimension2=Cm_aileron_wing_2  BreakpointsForDimension3=Cm_aileron_wing_3  BreakpointsForDimension4=Cm_aileron_wing_4  BreakpointsForDimension5=Cm_aileron_wing_5  BreakpointsForDimension6=Cm_aileron_wing_6  BreakpointsForDimension7=Cm_aileron_wing_7  Table=Cm_aileron_wing_val  InternalRulePriority=Speed  OutDataTypeStr=Inherit: Inherit via back propagation  RndMeth=Simplest
      settings: InputPortMap=u0,u1,u2,u3,u4,u5,u6
  n-D Lookup Table54 : Lookup_n-D  NumberOfTableDimensions=6  BreakpointsForDimension1=Cm_tail_1  BreakpointsForDimension2=Cm_tail_2  BreakpointsForDimension3=Cm_tail_3  BreakpointsForDimension4=Cm_tail_4  BreakpointsForDimension5=Cm_tail_5  BreakpointsForDimension6=Cm_tail_6  BreakpointsForDimension7=CX_tail_7  Table=Cm_tail_val  InternalRulePriority=Speed  OutDataTypeStr=Inherit: Inherit via back propagation  RndMeth=Simplest
      settings: InputPortMap=u0,u1,u2,u3,u4,u5
  n-D Lookup Table55 : Lookup_n-D  NumberOfTableDimensions=6  BreakpointsForDimension1=Cm_tail_damp_p_1  BreakpointsForDimension2=Cm_tail_damp_p_2  BreakpointsForDimension3=Cm_tail_damp_p_3  BreakpointsForDimension4=Cm_tail_damp_p_4  BreakpointsForDimension5=Cm_tail_damp_p_5  BreakpointsForDimension6=Cm_tail_damp_p_6  BreakpointsForDimension7=CX_tail_7  Table=Cm_tail_damp_p_val  InternalRulePriority=Speed  OutDataTypeStr=Inherit: Inherit via back propagation  RndMeth=Simplest
      settings: InputPortMap=u0,u1,u2,u3,u4,u5
  n-D Lookup Table56 : Lookup_n-D  NumberOfTableDimensions=6  BreakpointsForDimension1=Cm_tail_damp_q_1  BreakpointsForDimension2=Cm_tail_damp_q_2  BreakpointsForDimension3=Cm_tail_damp_q_3  BreakpointsForDimension4=Cm_tail_damp_q_4  BreakpointsForDimension5=Cm_tail_damp_q_5  BreakpointsForDimension6=Cm_tail_damp_q_6  BreakpointsForDimension7=CX_tail_7  Table=Cm_tail_damp_q_val  InternalRulePriority=Speed  OutDataTypeStr=Inherit: Inherit via back propagation  RndMeth=Simplest
      settings: InputPortMap=u0,u1,u2,u3,u4,u5
  n-D Lookup Table57 : Lookup_n-D  NumberOfTableDimensions=6  BreakpointsForDimension1=Cm_tail_damp_r_1  BreakpointsForDimension2=Cm_tail_damp_r_2  BreakpointsForDimension3=Cm_tail_damp_r_3  BreakpointsForDimension4=Cm_tail_damp_r_4  BreakpointsForDimension5=Cm_tail_damp_r_5  BreakpointsForDimension6=Cm_tail_damp_r_6  BreakpointsForDimension7=CX_tail_7  Table=Cm_tail_damp_r_val  InternalRulePriority=Speed  OutDataTypeStr=Inherit: Inherit via back propagation  RndMeth=Simplest
      settings: InputPortMap=u0,u1,u2,u3,u4,u5
  n-D Lookup Table58 : Lookup_n-D  NumberOfTableDimensions=6  BreakpointsForDimension1=Cm_wing_1  BreakpointsForDimension2=Cm_wing_2  BreakpointsForDimension3=Cm_wing_3  BreakpointsForDimension4=Cm_wing_4  BreakpointsForDimension5=Cm_wing_5  BreakpointsForDimension6=Cm_wing_6  BreakpointsForDimension7=CX_flap_wing_7  Table=Cm_wing_val  InternalRulePriority=Speed  OutDataTypeStr=Inherit: Inherit via back propagation  RndMeth=Simplest
      settings: InputPortMap=u0,u1,u2,u3,u4,u5
  n-D Lookup Table59 : Lookup_n-D  NumberOfTableDimensions=6  BreakpointsForDimension1=Cm_wing_damp_p_1  BreakpointsForDimension2=Cm_wing_damp_p_2  BreakpointsForDimension3=Cm_wing_damp_p_3  BreakpointsForDimension4=Cm_wing_damp_p_4  BreakpointsForDimension5=Cm_wing_damp_p_5  BreakpointsForDimension6=Cm_wing_damp_p_6  BreakpointsForDimension7=CX_flap_wing_7  Table=Cm_wing_damp_p_val  InternalRulePriority=Speed  OutDataTypeStr=Inherit: Inherit via back propagation  RndMeth=Simplest
      settings: InputPortMap=u0,u1,u2,u3,u4,u5
  Out1 : Outport
  wires:
  Matrix Multiply48/1 -> Add5/1
  MATLAB Function32/1(Cm_Scale_2) -> Product61/2
  n-D Lookup Table52/1 -> Mux51/2
  MATLAB Function62/1(Cm_Scale_7) -> Product68/2
  Cm_wing_damp_r/1(interp_point_1) -> n-D Lookup Table51/1
  Constant64/1 -> Mux51/1
  Cm_tail/4(interp_point_4) -> n-D Lookup Table54/4
  Cm_tail/3(interp_point_3) -> n-D Lookup Table54/3
  Constant63/1 -> Mux50/1
  Cm_wing_damp_q/5(interp_point_5) -> n-D Lookup Table50/5
  Cm_tail_damp_r/4(interp_point_4) -> n-D Lookup Table57/4
  MATLAB Function164/1(Tail_Transform) -> Matrix Multiply54/1
  Cm_rudder_tail/7(interp_point_7) -> n-D Lookup Table48/7
  Cm_wing_damp_q/3(interp_point_3) -> n-D Lookup Table50/3
  Matrix Multiply55/1 -> Add5/8
  Matrix Multiply59/1 -> Add5/12
  Cm_tail/5(interp_point_5) -> n-D Lookup Table54/5
  Cm_aileron_wing/5(interp_point_5) -> n-D Lookup Table53/5
  u/1 -> MATLAB Function62/1(u), Cm_tail_damp_r/1(u), MATLAB Function63/1(u), MATLAB Function156/1(u), Cm_wing/1(u), MATLAB Function36/1(u), MATLAB Function157/1(u), Cm_wing_damp_p/1(u), MATLAB Function64/1(u), MATLAB Function158/1(u), Cm_wing_damp_q/1(u), MATLAB Function65/1(u), MATLAB Function159/1(u), Cm_wing_damp_r/1(u), MATLAB Function66/1(u), Cm_hover_fuse/1(u), MATLAB Function77/1(u), MATLAB Function165/1(u), MATLAB Function164/1(u), MATLAB Function61/1(u), Cm_tail_damp_p/1(u), MATLAB Function163/1(u), MATLAB Function35/1(u), Cm_tail/1(u), MATLAB Function162/1(u), MATLAB Function34/1(u), Cm_rudder_tail/1(u), MATLAB Function161/1(u), MATLAB Function33/1(u), Cm_flap_wing/1(u), MATLAB Function155/1(u), MATLAB Function32/1(u), Cm_elevator_tail/1(u), MATLAB Function160/1(u), MATLAB Function31/1(u), Cm_aileron_wing/1(u), MATLAB Function154/1(u), Cm_tail_damp_q/1(u)
  Constant60/1 -> Mux58/1
  Mux57/1 -> Product69/1
  Matrix Multiply54/1 -> Add5/7
  MATLAB Function158/1(Wing_Transform) -> Matrix Multiply58/1
  n-D Lookup Table56/1 -> Mux56/2
  Constant144/1 -> Mux106/3
  Constant145/1 -> Mux106/1
  Mux61/1 -> Product63/1
  Product71/1 -> Matrix Multiply57/2
  MATLAB Function77/1(Cm_Scale_13) -> Product104/2
  Matrix Multiply58/1 -> Add5/11
  Cm_wing_damp_r/3(interp_point_3) -> n-D Lookup Table51/3
  Cm_wing_damp_p/5(interp_point_5) -> n-D Lookup Table59/5
  Cm_wing_damp_q/1(interp_point_1) -> n-D Lookup Table50/1
  Mux54/1 -> Product66/1
  Cm_tail_damp_q/4(interp_point_4) -> n-D Lookup Table56/4
  Cm_elevator_tail/2(interp_point_2) -> n-D Lookup Table52/2
  Cm_wing_damp_p/1(interp_point_1) -> n-D Lookup Table59/1
  Product70/1 -> Matrix Multiply56/2
  Cm_wing_damp_q/2(interp_point_2) -> n-D Lookup Table50/2
  Cm_elevator_tail/4(interp_point_4) -> n-D Lookup Table52/4
  Product61/1 -> Matrix Multiply49/2
  Mux56/1 -> Product68/1
  Matrix Multiply50/1 -> Add5/3
  n-D Lookup Table54/1 -> Mux54/2
  Mux51/1 -> Product61/1
  Cm_wing/6(interp_point_6) -> n-D Lookup Table58/6
  Cm_tail_damp_p/1(interp_point_1) -> n-D Lookup Table55/1
  Constant69/1 -> Mux56/1
  Product63/1 -> Matrix Multiply59/2
  Cm_flap_wing/7(interp_point_7) -> n-D Lookup Table49/7
  Constant70/1 -> Mux57/1
  n-D Lookup Table50/1 -> Mux60/2
  n-D Lookup Table51/1 -> Mux61/2
  MATLAB Function31/1(Cm_Scale_1) -> Product60/2
  Matrix Multiply52/1 -> Add5/5
  Cm_elevator_tail/5(interp_point_5) -> n-D Lookup Table52/5
  MATLAB Function33/1(Cm_Scale_3) -> Product64/2
  Product67/1 -> Matrix Multiply53/2
  n-D Lookup Table104/1 -> Mux106/2
  Constant55/1 -> Mux54/3
  Constant61/1 -> Mux60/3
  Matrix Multiply51/1 -> Add5/4
  n-D Lookup Table48/1 -> Mux53/2
  Cm_rudder_tail/2(interp_point_2) -> n-D Lookup Table48/2
  MATLAB Function34/1(Cm_Scale_4) -> Product65/2
  Product104/1 -> Add5/13
  Cm_tail_damp_r/2(interp_point_2) -> n-D Lookup Table57/2
  Cm_flap_wing/5(interp_point_5) -> n-D Lookup Table49/5
  Cm_hover_fuse/3(interp_point_3) -> n-D Lookup Table104/3
  Cm_tail_damp_q/5(interp_point_5) -> n-D Lookup Table56/5
  Cm_aileron_wing/6(interp_point_6) -> n-D Lookup Table53/6
  Cm_tail_damp_p/6(interp_point_6) -> n-D Lookup Table55/6
  Constant57/1 -> Mux56/3
  n-D Lookup Table58/1 -> Mux58/2
  Constant72/1 -> Mux59/1
  MATLAB Function165/1(Tail_Transform) -> Matrix Multiply55/1
  n-D Lookup Table57/1 -> Mux57/2
  Cm_wing/2(interp_point_2) -> n-D Lookup Table58/2
  Constant58/1 -> Mux57/3
  Constant73/1 -> Mux61/3
  Cm_wing_damp_p/3(interp_point_3) -> n-D Lookup Table59/3
  Cm_wing/1(interp_point_1) -> n-D Lookup Table58/1
  Matrix Multiply57/1 -> Add5/10
  Cm_wing_damp_r/6(interp_point_6) -> n-D Lookup Table51/6
  Constant52/1 -> Mux51/3
  Add5/1 -> Out1/1
  Cm_elevator_tail/3(interp_point_3) -> n-D Lookup Table52/3
  Cm_wing_damp_p/2(interp_point_2) -> n-D Lookup Table59/2
  MATLAB Function65/1(Cm_Scale_11) -> Product62/2
  Product66/1 -> Matrix Multiply52/2
  MATLAB Function64/1(Cm_Scale_10) -> Product71/2
  Mux106/1 -> Product104/1
  Cm_rudder_tail/4(interp_point_4) -> n-D Lookup Table48/4
  Constant62/1 -> Mux60/1
  Cm_rudder_tail/5(interp_point_5) -> n-D Lookup Table48/5
  Constant74/1 -> Mux61/1
  Constant51/1 -> Mux50/3
  Cm_elevator_tail/6(interp_point_6) -> n-D Lookup Table52/6
  Cm_tail/6(interp_point_6) -> n-D Lookup Table54/6
  Cm_wing_damp_q/6(interp_point_6) -> n-D Lookup Table50/6
  Cm_tail_damp_q/2(interp_point_2) -> n-D Lookup Table56/2
  Cm_flap_wing/2(interp_point_2) -> n-D Lookup Table49/2
  Cm_tail/2(interp_point_2) -> n-D Lookup Table54/2
  Cm_tail_damp_p/2(interp_point_2) -> n-D Lookup Table55/2
  Mux52/1 -> Product64/1
  n-D Lookup Table53/1 -> Mux50/2
  Constant53/1 -> Mux52/3
  Constant65/1 -> Mux52/1
  Mux50/1 -> Product60/1
  Constant66/1 -> Mux53/1
  Constant54/1 -> Mux53/3
  Constant68/1 -> Mux55/1
  Mux59/1 -> Product71/1
  Product62/1 -> Matrix Multiply58/2
  Product69/1 -> Matrix Multiply55/2
  Matrix Multiply49/1 -> Add5/2
  Matrix Multiply53/1 -> Add5/6
  Matrix Multiply56/1 -> Add5/9
  n-D Lookup Table55/1 -> Mux55/2
  Cm_tail_damp_q/1(interp_point_1) -> n-D Lookup Table56/1
  Cm_tail_damp_r/6(interp_point_6) -> n-D Lookup Table57/6
  Constant71/1 -> Mux59/3
  MATLAB Function35/1(Cm_Scale_5) -> Product66/2
  Cm_tail_damp_q/6(interp_point_6) -> n-D Lookup Table56/6
  Constant56/1 -> Mux55/3
  MATLAB Function163/1(Tail_Transform) -> Matrix Multiply53/1
  Product60/1 -> Matrix Multiply48/2
  n-D Lookup Table59/1 -> Mux59/2
  MATLAB Function61/1(Cm_Scale_6) -> Product67/2
  MATLAB Function66/1(Cm_Scale_12) -> Product63/2
  Cm_wing_damp_p/6(interp_point_6) -> n-D Lookup Table59/6
  Cm_wing_damp_r/4(interp_point_4) -> n-D Lookup Table51/4
  Cm_wing_damp_r/2(interp_point_2) -> n-D Lookup Table51/2
  Cm_flap_wing/6(interp_point_6) -> n-D Lookup Table49/6
  Cm_tail_damp_p/4(interp_point_4) -> n-D Lookup Table55/4
  Cm_rudder_tail/3(interp_point_3) -> n-D Lookup Table48/3
  Cm_flap_wing/1(interp_point_1) -> n-D Lookup Table49/1
  Cm_wing/4(interp_point_4) -> n-D Lookup Table58/4
  Cm_wing_damp_q/4(interp_point_4) -> n-D Lookup Table50/4
  Cm_flap_wing/4(interp_point_4) -> n-D Lookup Table49/4
  Cm_wing/5(interp_point_5) -> n-D Lookup Table58/5
  Cm_aileron_wing/1(interp_point_1) -> n-D Lookup Table53/1
  MATLAB Function63/1(Cm_Scale_8) -> Product69/2
  Constant67/1 -> Mux54/1
  Cm_wing_damp_r/5(interp_point_5) -> n-D Lookup Table51/5
  Cm_rudder_tail/1(interp_point_1) -> n-D Lookup Table48/1
  Cm_aileron_wing/3(interp_point_3) -> n-D Lookup Table53/3
  Cm_rudder_tail/6(interp_point_6) -> n-D Lookup Table48/6
  Cm_elevator_tail/1(interp_point_1) -> n-D Lookup Table52/1
  Cm_tail_damp_r/1(interp_point_1) -> n-D Lookup Table57/1
  Cm_tail_damp_r/3(interp_point_3) -> n-D Lookup Table57/3
  Cm_flap_wing/3(interp_point_3) -> n-D Lookup Table49/3
  Cm_wing_damp_p/4(interp_point_4) -> n-D Lookup Table59/4
  Cm_tail/1(interp_point_1) -> n-D Lookup Table54/1
  Cm_tail_damp_p/5(interp_point_5) -> n-D Lookup Table55/5
  MATLAB Function160/1(Tail_Transform) -> Matrix Multiply49/1
  Mux55/1 -> Product67/1
  Mux58/1 -> Product70/1
  Mux60/1 -> Product62/1
  Mux53/1 -> Product65/1
  Cm_hover_fuse/1(interp_point_1) -> n-D Lookup Table104/1
  Cm_aileron_wing/4(interp_point_4) -> n-D Lookup Table53/4
  MATLAB Function156/1(Wing_Transform) -> Matrix Multiply56/1
  MATLAB Function36/1(Cm_Scale_9) -> Product70/2
  Cm_aileron_wing/7(interp_point_7) -> n-D Lookup Table53/7
  MATLAB Function162/1(Tail_Transform) -> Matrix Multiply52/1
  Cm_tail_damp_r/5(interp_point_5) -> n-D Lookup Table57/5
  Cm_tail_damp_q/3(interp_point_3) -> n-D Lookup Table56/3
  MATLAB Function154/1(Wing_Transform) -> Matrix Multiply48/1
  MATLAB Function157/1(Wing_Transform) -> Matrix Multiply57/1
  Constant59/1 -> Mux58/3
  Product65/1 -> Matrix Multiply51/2
  Product64/1 -> Matrix Multiply50/2
  MATLAB Function159/1(Wing_Transform) -> Matrix Multiply59/1
  MATLAB Function161/1(Tail_Transform) -> Matrix Multiply51/1
  Product68/1 -> Matrix Multiply54/2
  Cm_aileron_wing/2(interp_point_2) -> n-D Lookup Table53/2
  Cm_hover_fuse/2(interp_point_2) -> n-D Lookup Table104/2
  n-D Lookup Table49/1 -> Mux52/2
  Cm_wing/3(interp_point_3) -> n-D Lookup Table58/3
  Cm_tail_damp_p/3(interp_point_3) -> n-D Lookup Table55/3
  MATLAB Function155/1(Wing_Transform) -> Matrix Multiply50/1
  Cm_elevator_tail/7(interp_point_7) -> n-D Lookup Table52/7
